simulink model "EcmoDevice"  (R2019b)
settings: Solver=VariableStepAuto  StartTime=0.0  StopTime=10.0  RelTol=1e-3
values from neighbouring files (symbols this model uses):
  alpha1 = 0.03198    [xFinalDisease.m]
  alpha2 = 0.05591    [xFinalDisease.m]
  beta1 = 0.008275    [xFinalDisease.m]
  beta2 = 0.03255    [xFinalDisease.m]
  CsatCO2 = 1.9488    [xFinalDisease.m]
  CsatO2 = 0.2128    [xFinalDisease.m]
  h1 = 0.3836    [xFinalDisease.m]
  h2 = 1.819    [xFinalDisease.m]
  K1 = 15.0    (= 15)    [xFinalDisease.m]
  K2 = 194.4    [xFinalDisease.m]
  Patm = 760.0    (= 760)    [xFinalDisease.m]
  Pws = 47.0    (= 47)    [xFinalDisease.m]
  Tsamp = 1e-3    (= 0.001)    [xFinalDisease.m]
undefined symbols (not defined in the file or in its folder): FIEO2, JL, kem, PECO2_IC, PEO2_IC, R, VECO2, VEO2
libraries: fl_lib x9, nesl_utility x3, simulink x2
settings Model: Creator=SÜLEYMAN  LastModifiedBy=SÜLEYMAN

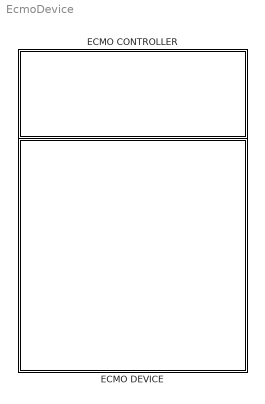
== system EcmoDevice ==
  ECMO CONTROLLER : Subsystem
  ECMO DEVICE : Subsystem

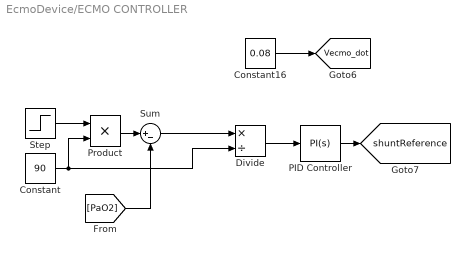
== system EcmoDevice/ECMO CONTROLLER ==
  Constant : Constant  Value=90
  Constant16 : Constant  Value=0.08
  Divide : Product  Inputs=*/
  PID Controller : simulink/Continuous/PID Controller  Controller=PI  Form=Parallel  TimeDomain=Continuous-time  SampleTime=-1  IntegratorMethod=Forward Euler  FilterMethod=Forward Euler  ControllerParametersSource=internal  P=10  I=4  D=600  UseFilter=on  N=100  TunerSelectOption=Transfer Function Based (PID Tuner App)  InitialConditionSource=internal  InitialConditionForIntegrator=0  InitialConditionForFilter=0  DifferentiatorICPrevScaledInput=0  ExternalReset=none  TrackingMode=off  Kt=1  LimitOutput=on  UpperSaturationLimit=1  LowerSaturationLimit=0  LinearizeAsGain=on  AntiWindupMode=none  Kb=1  POutMin=[]  POutMax=[]  IOutMin=[]  IOutMax=[]  DOutMin=[]  DOutMax=[]  NOutMin=[]  NOutMax=[]  SumOutMin=[]  SumOutMax=[]  SaturationOutMin=[]  SaturationOutMax=[]  PParamMin=[]  PParamMax=[]  IParamMin=[]  IParamMax=[]  DParamMin=[]  DParamMax=[]  NParamMin=[]  NParamMax=[]  KbParamMin=[]  KbParamMax=[]  KtParamMin=[]  KtParamMax=[]  KbOutMin=[]  KbOutMax=[]  KtOutMin=[]  KtOutMax=[]  IntegratorOutMin=[]  IntegratorOutMax=[]  FilterOutMin=[]  FilterOutMax=[]  SumI1OutMin=[]  SumI1OutMax=[]  SumI2OutMin=[]  SumI2OutMax=[]  SumI3OutMin=[]  SumI3OutMax=[]  SumI4OutMin=[]  SumI4OutMax=[]  SumDOutMin=[]  SumDOutMax=[]  DifferentiatorOutMin=[]  DifferentiatorOutMax=[]  FilterDiffOutCoefMin=[]  FilterDiffOutCoefMax=[]  ReciprocalOutMin=[]  ReciprocalOutMax=[]  SumDenOutMin=[]  SumDenOutMax=[]  SumNumOutMin=[]  SumNumOutMax=[]  DivideOutMin=[]  DivideOutMax=[]  IntegratorContinuousStateAttributes=''  IntegratorStateMustResolveToSignalObject=off  IntegratorRTWStateStorageClass=Auto  FilterContinuousStateAttributes=''  FilterStateMustResolveToSignalObject=off  FilterRTWStateStorageClass=Auto  ParallelPVariant=InternalParameters  IdealPVariant=Disabled  IVariant=InternalParameters  DVariant=Disabled  IntegratorVariant=Continuous  SatVariant=Enabled  AWVariant=Passthrough  PCopyVariant=Disabled  TRVariant=Disabled  FdbkBlocksVariant=Forward  IdealPFdbkVariant=Disabled  SatFdbkVariant=Disabled  DerivativeFilterVariant=Disabled  NVariant=Disabled  NCopyVariant=Disabled_SignalSpec  FilterICVariant=Disabled  IntegratorICVariant=InternalICs  ExternalResetVariant=Disabled  TRSumVariant=Passthrough  SumFdbkVariant=Disabled  SumVariant=Sum_PI
  Product : Product
  Step : Step  Time=0  SampleTime=0
  Sum : Sum  Inputs=|+-
  tag scope: Vecmo_dot=global, shuntReference=global
  wires:
  Product/1 -> Sum/1
  [PaO2] -> Sum/2
  PID Controller/1 -> [shuntReference]
  Constant16/1 -> [Vecmo_dot]
  Sum/1 -> Divide/1
  Divide/1 -> PID Controller/1
  Constant/1 -> Divide/2, Product/2
  Step/1 -> Product/1

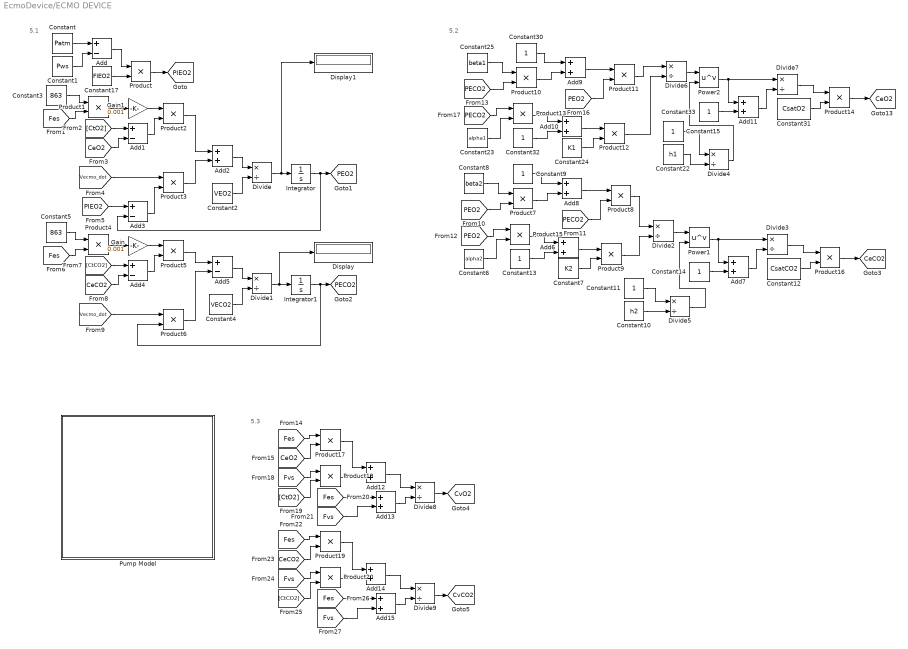
== system EcmoDevice/ECMO DEVICE ==
  note: 5.3
  note: 5.1
  note: 5.2
  Add{,1,3..5} (5 alike) : Sum  Inputs=+-
  Add{2,6..15} (11 alike) : Sum
  Constant : Constant  Value=Patm
  Constant1 : Constant  Value=Pws
  Constant10 : Constant  Value=h2  SampleTime=Tsamp
  Constant{9,11,13..15,30,32..33} (8 alike) : Constant  SampleTime=Tsamp
  Constant12 : Constant  Value=CsatCO2  SampleTime=Tsamp
  Constant17 : Constant  Value=FIEO2
  Constant2 : Constant  Value=VEO2
  Constant22 : Constant  Value=h1  SampleTime=Tsamp
  Constant23 : Constant  Value=alpha1  SampleTime=Tsamp
  Constant24 : Constant  Value=K1  SampleTime=Tsamp
  Constant25 : Constant  Value=beta1  SampleTime=Tsamp
  Constant3 : Constant  Value=863
  Constant31 : Constant  Value=CsatO2  SampleTime=Tsamp
  Constant4 : Constant  Value=VECO2
  Constant5 : Constant  Value=863
  Constant6 : Constant  Value=alpha2  SampleTime=Tsamp
  Constant7 : Constant  Value=K2  SampleTime=Tsamp
  Constant8 : Constant  Value=beta2  SampleTime=Tsamp
  Display : Display
  Display1 : Display
  Divide{,1..9} (10 alike) : Product  Inputs=*/
  Gain : Gain  Gain=0.001
  Gain1 : Gain  Gain=0.001
  Integrator : Integrator  InitialCondition=PEO2_IC
  Integrator1 : Integrator  InitialCondition=PECO2_IC
  Power1 : Math  Operator=pow  SignedPower=off  SaturateOnIntegerOverflow=on
  Power2 : Math  Operator=pow  SignedPower=off  SaturateOnIntegerOverflow=on
  Product{,1..20} (21 alike) : Product
  "Pump Model " : Subsystem
  tag scope: CeCO2=global, CeO2=global, CvCO2=global, CvO2=global, PECO2=global, PEO2=global, PIEO2=global
  wires:
  [PECO2] -> Product8/2
  Constant2/1 -> Divide/2
  Product11/1 -> Divide6/1
  Divide4/1 -> Power2/2
  Constant15/1 -> Divide4/1
  Product7/1 -> Add8/2
  [Fes] -> Add13/1
  Add12/1 -> Divide8/1
  Gain/1 -> Product5/1
  Constant13/1 -> Add6/2
  Product20/1 -> Add14/2
  [Fvs] -> Add15/2
  [Fes] -> Product19/1
  Constant3/1 -> Product1/1
  [Fes] -> Product17/1
  [PECO2] -> Product10/2
  Power1/1 -> Add7/1, Divide3/1
  Add2/1 -> Divide/1
  Constant10/1 -> Divide5/2
  Add13/1 -> Divide8/2
  [CtO2] -> Product18/2
  Divide6/1 -> Power2/1
  Add3/1 -> Product3/2
  [PEO2] -> Product11/2
  Add10/1 -> Product12/1
  Divide1/1 -> Display/1, Integrator1/1
  [Fes] -> Product1/2
  Constant24/1 -> Product12/2
  Integrator1/1 -> Product6/2, [PECO2]
  Constant1/1 -> Add/2
  Constant6/1 -> Product15/2
  Integrator/1 -> Add3/2, [PEO2]
  Add11/1 -> Divide7/2
  Product8/1 -> Divide2/1
  Product17/1 -> Add12/1
  [Vecmo_dot] -> Product3/1
  [CtCO2] -> Add4/1
  Constant7/1 -> Product9/2
  Product18/1 -> Add12/2
  Product10/1 -> Add9/2
  Product14/1 -> [CeO2]
  Add4/1 -> Product5/2
  [PIEO2] -> Add3/1
  Product6/1 -> Add5/2
  Constant14/1 -> Add7/2
  Divide5/1 -> Power1/2
  Gain1/1 -> Product2/1
  Add9/1 -> Product11/1
  Product5/1 -> Add5/1
  Constant33/1 -> Add11/2
  Add15/1 -> Divide9/2
  Add8/1 -> Product8/1
  Constant11/1 -> Divide5/1
  [PEO2] -> Product15/1
  Constant5/1 -> Product4/1
  Constant17/1 -> Product/2
  Constant31/1 -> Product14/2
  Divide3/1 -> Product16/1
  Divide/1 -> Display1/1, Integrator/1
  Add1/1 -> Product2/2
  Add7/1 -> Divide3/2
  Add/1 -> Product/1
  Constant/1 -> Add/1
  Power2/1 -> Add11/1, Divide7/1
  Add5/1 -> Divide1/1
  Constant12/1 -> Product16/2
  Product9/1 -> Divide2/2
  Product16/1 -> [CeCO2]
  Constant32/1 -> Add10/2
  Product12/1 -> Divide6/2
  Product3/1 -> Add2/2
  Divide2/1 -> Power1/1
  [Fvs] -> Product18/1
  [CeCO2] -> Product19/2
  [Fes] -> Product4/2
  Add14/1 -> Divide9/1
  Divide8/1 -> [CvO2]
  Constant9/1 -> Add8/1
  [CtO2] -> Add1/1
  [Fvs] -> Add13/2
  Divide7/1 -> Product14/1
  Constant4/1 -> Divide1/2
  Divide9/1 -> [CvCO2]
  Constant8/1 -> Product7/1
  Add6/1 -> Product9/1
  Product1/1 -> Gain1/1
  Constant30/1 -> Add9/1
  Product2/1 -> Add2/1
  Product15/1 -> Add6/1
  Product/1 -> [PIEO2]
  Constant25/1 -> Product10/1
  [PECO2] -> Product13/1
  Constant23/1 -> Product13/2
  [CeO2] -> Product17/2
  Product4/1 -> Gain/1
  Product13/1 -> Add10/1
  [Fvs] -> Product20/1
  Constant22/1 -> Divide4/2
  [CeO2] -> Add1/2
  [PEO2] -> Product7/2
  [Vecmo_dot] -> Product6/1
  [CeCO2] -> Add4/2
  [CtCO2] -> Product20/2
  [Fes] -> Add15/1
  Product19/1 -> Add14/1

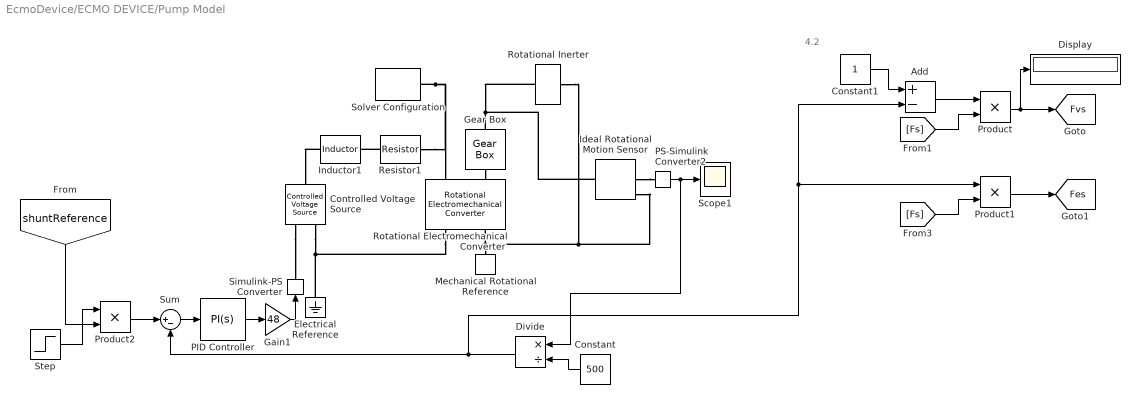
== system EcmoDevice/ECMO DEVICE/Pump Model  ==
  note: 4.2
  Add : Sum  Inputs=+-
  Constant : Constant  Value=500
  Constant1 : Constant
  Controlled Voltage Source : fl_lib/Electrical/Electrical Sources/Controlled Voltage Source
  Display : Display
  Divide : Product  Inputs=*/
  Electrical Reference : fl_lib/Electrical/Electrical Elements/Electrical Reference
  Gain1 : Gain  Gain=48
  Gear Box : fl_lib/Mechanical/Mechanisms/Gear Box  ratio=Ng  t_in_specify=off  t_in_priority=None  t_in=0 N*m  t_in_nominal_specify=off  t_in_nominal_unit=N*m  t_in_nominal_value=1  t_out_specify=off  t_out_priority=None  t_out=0 N*m  t_out_nominal_specify=off  t_out_nominal_unit=N*m  t_out_nominal_value=1
  Ideal Rotational Motion Sensor : fl_lib/Mechanical/Mechanical Sensors/Ideal Rotational Motion Sensor  offset=0 rad
  Inductor1 : fl_lib/Electrical/Electrical Elements/Inductor  l=L mH  r=0 Ohm  g=1e-9 1/Ohm  i_specify=off  i_priority=None  i=0 A  i_nominal_specify=off  i_nominal_unit=A  i_nominal_value=1  v_specify=off  v_priority=None  v=0 V  v_nominal_specify=off  v_nominal_unit=V  v_nominal_value=1  i_L_specify=off  i_L_priority=High  i_L=0 A  i_L_nominal_specify=off  i_L_nominal_unit=A  i_L_nominal_value=1
  Mechanical Rotational Reference : fl_lib/Mechanical/Rotational Elements/Mechanical Rotational Reference
  PID Controller : simulink/Continuous/PID Controller  Controller=PI  Form=Parallel  TimeDomain=Continuous-time  SampleTime=-1  IntegratorMethod=Forward Euler  FilterMethod=Forward Euler  ControllerParametersSource=internal  P=300  I=48.35  D=0  UseFilter=on  N=100  TunerSelectOption=Transfer Function Based (PID Tuner App)  InitialConditionSource=internal  InitialConditionForIntegrator=0  InitialConditionForFilter=0  DifferentiatorICPrevScaledInput=0  ExternalReset=none  TrackingMode=off  Kt=1  LimitOutput=on  UpperSaturationLimit=1  LowerSaturationLimit=0  LinearizeAsGain=on  AntiWindupMode=none  Kb=1  POutMin=[]  POutMax=[]  IOutMin=[]  IOutMax=[]  DOutMin=[]  DOutMax=[]  NOutMin=[]  NOutMax=[]  SumOutMin=[]  SumOutMax=[]  SaturationOutMin=[]  SaturationOutMax=[]  PParamMin=[]  PParamMax=[]  IParamMin=[]  IParamMax=[]  DParamMin=[]  DParamMax=[]  NParamMin=[]  NParamMax=[]  KbParamMin=[]  KbParamMax=[]  KtParamMin=[]  KtParamMax=[]  KbOutMin=[]  KbOutMax=[]  KtOutMin=[]  KtOutMax=[]  IntegratorOutMin=[]  IntegratorOutMax=[]  FilterOutMin=[]  FilterOutMax=[]  SumI1OutMin=[]  SumI1OutMax=[]  SumI2OutMin=[]  SumI2OutMax=[]  SumI3OutMin=[]  SumI3OutMax=[]  SumI4OutMin=[]  SumI4OutMax=[]  SumDOutMin=[]  SumDOutMax=[]  DifferentiatorOutMin=[]  DifferentiatorOutMax=[]  FilterDiffOutCoefMin=[]  FilterDiffOutCoefMax=[]  ReciprocalOutMin=[]  ReciprocalOutMax=[]  SumDenOutMin=[]  SumDenOutMax=[]  SumNumOutMin=[]  SumNumOutMax=[]  DivideOutMin=[]  DivideOutMax=[]  IntegratorContinuousStateAttributes=''  IntegratorStateMustResolveToSignalObject=off  IntegratorRTWStateStorageClass=Auto  FilterContinuousStateAttributes=''  FilterStateMustResolveToSignalObject=off  FilterRTWStateStorageClass=Auto  ParallelPVariant=InternalParameters  IdealPVariant=Disabled  IVariant=InternalParameters  DVariant=Disabled  IntegratorVariant=Continuous  SatVariant=Enabled  AWVariant=Passthrough  PCopyVariant=Disabled  TRVariant=Disabled  FdbkBlocksVariant=Forward  IdealPFdbkVariant=Disabled  SatFdbkVariant=Disabled  DerivativeFilterVariant=Disabled  NVariant=Disabled  NCopyVariant=Disabled_SignalSpec  FilterICVariant=Disabled  IntegratorICVariant=InternalICs  ExternalResetVariant=Disabled  TRSumVariant=Passthrough  SumFdbkVariant=Disabled  SumVariant=Sum_PI
  PS-Simulink Converter2 : nesl_utility/PS-Simulink Converter  PhysicalDomain=network_engine_domain  SubClassName=ps_output  LeftPortType=input  RightPortType=output  PseudoPeriodic=off  Frequencies=[]  Unit=inherit  AffineConversion=off
  Product : Product
  Product1 : Product
  Product2 : Product
  Resistor1 : fl_lib/Electrical/Electrical Elements/Resistor  R=R Ohm  i_specify=off  i_priority=None  i=0 A  i_nominal_specify=off  i_nominal_unit=A  i_nominal_value=1  v_specify=off  v_priority=None  v=0 V  v_nominal_specify=off  v_nominal_unit=V  v_nominal_value=1
  Rotational Electromechanical Converter : fl_lib/Electrical/Electrical Elements/Rotational Electromechanical Converter  K=kem V/(rad/s)  i_specify=off  i_priority=None  i=0 A  i_nominal_specify=off  i_nominal_unit=A  i_nominal_value=1  v_specify=off  v_priority=None  v=0 V  v_nominal_specify=off  v_nominal_unit=V  v_nominal_value=1  t_specify=off  t_priority=None  t=0 N*m  t_nominal_specify=off  t_nominal_unit=N*m  t_nominal_value=1  w_specify=off  w_priority=None  w=0 rad/s  w_nominal_specify=off  w_nominal_unit=rad/s  w_nominal_value=1
      settings: SourceProductName=Simscape
  Rotational Inerter : fl_lib/Mechanical/Rotational Elements/Rotational Inerter  B=JL kg*m^2  w_specify=off  w_priority=High  w=0 rad/s  w_nominal_specify=off  w_nominal_unit=rad/s  w_nominal_value=1  t_specify=off  t_priority=None  t=0 N*m  t_nominal_specify=off  t_nominal_unit=N*m  t_nominal_value=1
      settings: SourceProductName=Simscape  SourceProductBaseCode=SS  InternalSimscapePortConfiguration="{\"Bottom\":[],\"Left\":[{\"id\":\"R\",\"label\":\"R\",\"type\":\"foundation.mechanical.rotational.rotational\"}],\"Right\":[{\"id\":\"C\",\"label\":\"C\",\"type\":\"foundation.mechanical.rotational.rotational\"}],\"Top\":[]}"
  Scope1 : Scope
  Simulink-PS Converter : nesl_utility/Simulink-PS Converter  PhysicalDomain=network_engine_domain  SubClassName=ps_input  LeftPortType=input  RightPortType=output  PseudoPeriodic=off  Frequencies=[]  NoiseDistribution=none  NoiseParameters=[]  Unit=1  AffineConversion=off  FilteringAndDerivatives=provide  SimscapeFilterOrder=1  InputFilterTimeConstant=0.001  UdotUserProvided=0
  Solver Configuration : nesl_utility/Solver Configuration  PhysicalDomain=network_engine_domain  SubClassName=solver  LeftPortType=input  RightPortType=generic  Tones=[]  Harmonics=[]  SimulateNoise=off  Profile=off  UseLocalSampling=off  EnableSwitchedLinearOptims=on  FrequencyDomain=off  UseCCode=off  RelTol=0.001  AbsTol=1e-06  MinStep=1e-09  ToWorkspace=off  RevertToSquareIcSolve=off  NumHomotopyIterations=100  PhasorMode=off  PhasorModeNumHarmonics=1  DoDC=off  ResidualTolerance=1e-09  UseLocalSolver=off  LocalSolverChoice=NE_BACKWARD_EULER_ADVANCER  LocalSolverSampleTime=0.001  DoFixedCost=off  MaxNonlinIter=3  MaxModeIter=2  LinearAlgebra=auto  EquationFormulation=NE_TIME_EF  DelaysMemoryBudget=1024  AutomaticFiltering=on  FilteringTimeConstant=0.001  PartitionStorageMethod=AS_NEEDED  PartitionMemoryBudget=1024  PartitionMethod=ROBUST
  Step : Step  Time=0  SampleTime=0
  Sum : Sum  Inputs=|+-
  tag scope: Fes=global, Fvs=global
  wires:
  Sum/1 -> PID Controller/1
  Gain1/1 -> Simulink-PS Converter/1
  Constant/1 -> Divide/2
  PS-Simulink Converter2/1 -> Scope1/1, Divide/1
  Product2/1 -> Sum/1
  Step/1 -> Product2/1
  Divide/1 -> Product1/1, Add/2, Sum/2
  Constant1/1 -> Add/1
  Add/1 -> Product/1
  [Fs] -> Product/2
  Product/1 -> Display/1, [Fvs]
  PID Controller/1 -> Gain1/1
  [Fs] -> Product1/2
  Product1/1 -> [Fes]
  [shuntReference] -> Product2/2
  connections:
  Ideal Rotational Motion Sensor/RConn1 -- Mechanical Rotational Reference/LConn1 -- Rotational Electromechanical Converter/RConn2 -- Rotational Inerter/RConn1
  Controlled Voltage Source/RConn2 -- Rotational Electromechanical Converter/RConn1 -- Electrical Reference/LConn1
  Gear Box/LConn1 -- Rotational Electromechanical Converter/LConn2
  Gear Box/RConn1 -- Rotational Inerter/LConn1 -- Ideal Rotational Motion Sensor/LConn1
  Solver Configuration/RConn1 -- Resistor1/RConn1 -- Rotational Electromechanical Converter/LConn1
  Ideal Rotational Motion Sensor/RConn2 -- PS-Simulink Converter2/LConn1
  Inductor1/LConn1 -- Controlled Voltage Source/LConn1
  Controlled Voltage Source/RConn1 -- Simulink-PS Converter/RConn1
  Resistor1/LConn1 -- Inductor1/RConn1
